simulink model "Simulation_Model"  (R2019b)
settings: Solver=FixedStepAuto  StartTime=0.0  StopTime=50  MaxStep=1  RelTol=1e-7
values from neighbouring files (symbols this model uses):
  Door_c = 50    [main.m]
  Door_k = 1000    [main.m]
  Door_mass = 3    [main.m]
  Ini_v = 0    [main.m]
  Sample_time = 0.1    [main.m]    (also in manual_env_for_test_slx.m; test_tool_initialize.m)
libraries: SignalEditorBlockLib x1
settings Model: Creator=M156732  LastModifiedBy=yangy
settings DataIOCC: ReturnWorkspaceOutputs=off
settings DebuggingCC: ArithmeticOperatorsInVariantConditions=warning
settings SFSimCC: CustomCodeUndefinedFunction=UseInterfaceOnly
settings RTWCC: GenCodeOnly=on

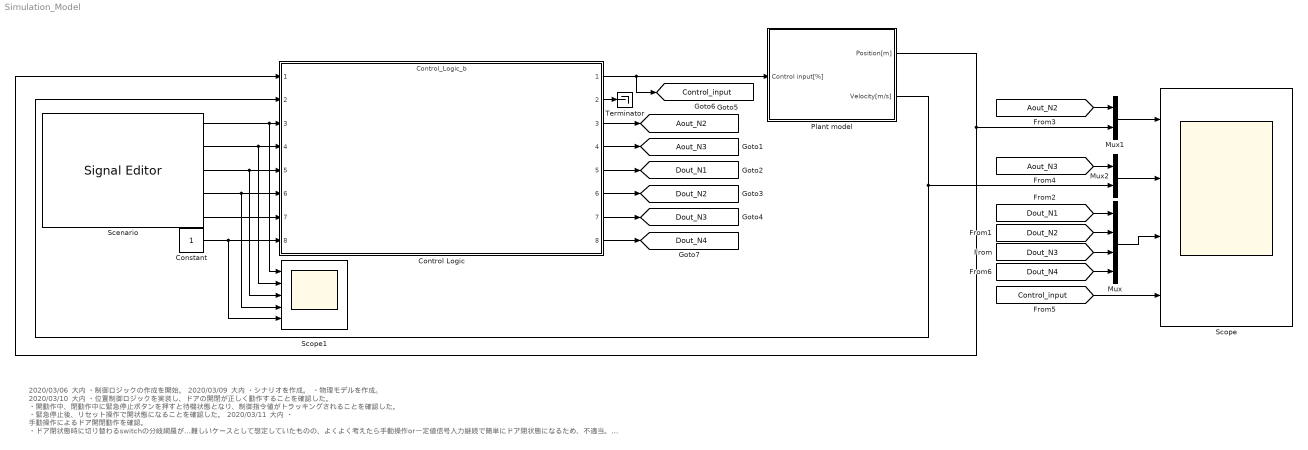
== system Simulation_Model ==
  note: 2020/03/06 大内
      | ・制御ロジックの作成を開始。
      | 2020/03/09 大内
      | ・シナリオを作成。
      | ・物理モデルを作成。
      | 2020/03/10 大内
      | ・位置制御ロジックを実装し、ドアの開閉が正しく動作することを確認した。
      | ・開動作中、閉動作中に緊急停止ボタンを押すと待機状態となり、制御指令値がトラッキングされることを確認した。
      | ・緊急停止後、リセット操作で開状態になることを確認した。
      | 2020/03/11 大内
      | ・ 手動操作によるドア開閉動作を確認。
      | ・ドア閉状態時に切り替わるswitchの分岐網羅が難しいケースとして想定していたものの、よくよく考えたら手動操作or一定値信号入力継続で簡単にドア閉状態になるため、不適当。
      | ドア閉状態になるには、① 通常動作によるドア開→ドア閉、②手動操作の2パターンを想定。そこで、a.人がドアの前に立ち、開いてから立ち去る or b.ドア開状態にならないとドアを閉め始めないと
      | いった条件を追加した。
      | 2020/03/12 大内
      | ・一旦ロジックは完成として、各POLの内部変数を変更したモデルを2つ作成した。
      | Logic_a：内部変数を0にして中身をいじれなくしたバージョン、
      | Logic_b：各々の内部変数を定義し、外部から変更を可能にしたバージョン
  Constant : Constant  OutDataTypeStr=boolean
  Control Logic : ModelReference  ModelNameDialog=Control_Logic_b.slx  SimulationMode=Normal  ModelReferenceVersion=1.275
  Mux : Mux
  Mux1 : Mux  Inputs=2
  Mux2 : Mux  Inputs=2
  Plant model : Subsystem
  Scenario : SignalEditorBlockLib/Signal Editor  FileName=Test_scenario.mat  ActiveScenario=Scenario2_DoorOpen_Close  ActiveSignal=Pressure  IsBus=off  OutputBusObjectStr=Bus: BusObject  SampleTime=Sample_time  Interpolate=off  ZeroCross=off  OutputAfterFinalValue=Setting to zero  Unit=kPa  PreserveSignalName=on
      settings: SourceProductName=Simulink
  Scope : Scope  NumInputPorts=4
  Scope1 : Scope  NumInputPorts=5
  Terminator : Terminator
  tag scope: Aout_N2=global, Aout_N3=global, Control_input=global, Dout_N1=global, Dout_N2=global, Dout_N3=global, Dout_N4=global
  wires:
  Control Logic/1 -> [Control_input], Plant model/1(Control input[%])
  Plant model/1(Position[m]) -> Mux1/2, Control Logic/1
  Plant model/2(Velocity[m/s]) -> Control Logic/2, Mux2/2
  Scenario/3 -> Scope1/3, Control Logic/5
  Control Logic/2 -> Terminator/1
  Scenario/1 -> Scope1/1, Control Logic/3
  [Dout_N2] -> Mux/2
  [Dout_N3] -> Mux/3
  [Dout_N1] -> Mux/1
  [Aout_N2] -> Mux1/1
  Mux1/1 -> Scope/1
  [Aout_N3] -> Mux2/1
  Mux2/1 -> Scope/2
  Mux/1 -> Scope/3
  [Control_input] -> Scope/4
  Scenario/2 -> Scope1/2, Control Logic/4
  Constant/1 -> Scope1/5, Control Logic/8
  Control Logic/3 -> [Aout_N2]
  Control Logic/4 -> [Aout_N3]
  Control Logic/5 -> [Dout_N1]
  Control Logic/6 -> [Dout_N2]
  Control Logic/7 -> [Dout_N3]
  Control Logic/8 -> [Dout_N4]
  [Dout_N4] -> Mux/4
  Scenario/4 -> Scope1/4, Control Logic/6
  Scenario/5 -> Control Logic/7

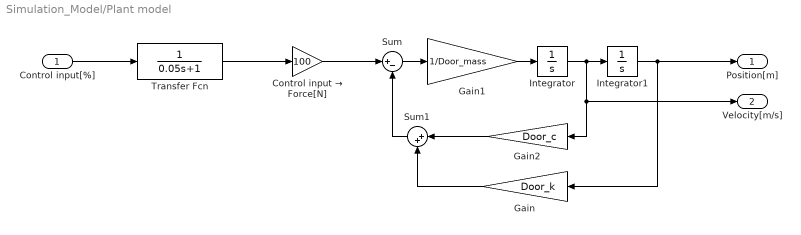
== system Simulation_Model/Plant model ==
  Control input[%] : Inport
  Control input → Force[N] : Gain  Gain=100
  Gain : Gain  Gain=Door_k
  Gain1 : Gain  Gain=1/Door_mass
  Gain2 : Gain  Gain=Door_c
  Integrator : Integrator  InitialCondition=Ini_v
  Integrator1 : Integrator
  Sum : Sum  Inputs=|+-
  Sum1 : Sum  Inputs=|++
  Transfer Fcn : TransferFcn  Denominator=[0.05 1]
  Position[m] : Outport  VectorParamsAs1DForOutWhenUnconnected=off
  Velocity[m/s] : Outport  Port=2  VectorParamsAs1DForOutWhenUnconnected=off
  wires:
  Control input[%]/1 -> Transfer Fcn/1
  Gain/1 -> Sum1/2
  Integrator/1 -> Velocity[m/s]/1, Gain2/1, Integrator1/1
  Sum/1 -> Gain1/1
  Gain2/1 -> Sum1/1
  Integrator1/1 -> Position[m]/1, Gain/1
  Gain1/1 -> Integrator/1
  Sum1/1 -> Sum/2
  Control input → Force[N]/1 -> Sum/1
  Transfer Fcn/1 -> Control input → Force[N]/1
